simulink model "dz1"  (R2023a)
settings: Solver=VariableStepAuto  StartTime=0.0  StopTime=10  RelTol=1e-3
settings Model: Creator=diontep  LastModifiedBy=diontep

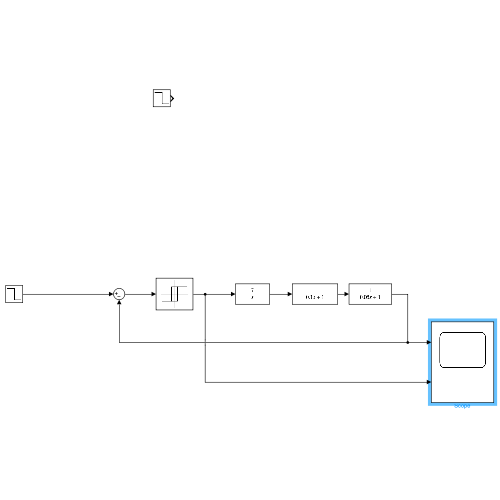
[thumbnail: Simulink's stored preview of the top-level diagram]
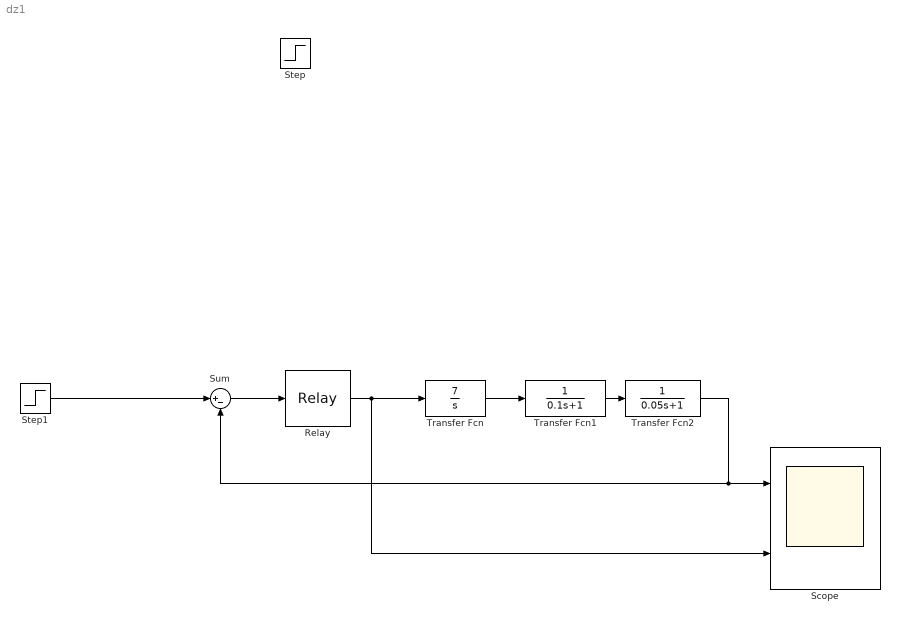
== system dz1 ==
  Relay : Relay  OnSwitchValue=1.5  OffSwitchValue=-1.5  OnOutputValue=12  OffOutputValue=-12
  Scope : Scope  NumInputPorts=2
  Step : Step  Before=5  After=0  SampleTime=0
  Step1 : Step  Before=5  After=0  SampleTime=0
  Sum : Sum  Inputs=|+-
  Transfer Fcn : TransferFcn  Numerator=[7]  Denominator=[1 0]
  Transfer Fcn1 : TransferFcn  Denominator=[0.1 1]
  Transfer Fcn2 : TransferFcn  Denominator=[0.05 1]
  wires:
  Step1/1 -> Sum/1
  Sum/1 -> Relay/1
  Relay/1 -> Scope/2, Transfer Fcn/1
  Transfer Fcn/1 -> Transfer Fcn1/1
  Transfer Fcn1/1 -> Transfer Fcn2/1
  Transfer Fcn2/1 -> Sum/2, Scope/1
